simulink model "MODAL"  (R2013a)
settings: Solver=ode45  StartTime=0.0  StopTime=10.0  RelTol=1e-3
undefined symbols (not defined in the file or in its folder): f, g1, g2, J, K, L, l1, l2, R
settings Model: Creator=ciottopinton_gus  LastModifiedBy=ciottopinton_gus

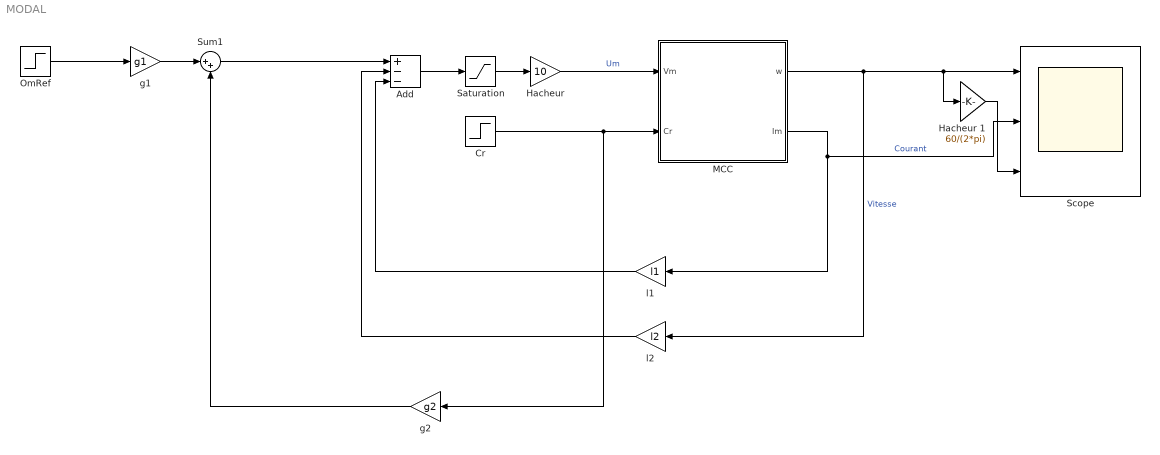
== system MODAL ==
  Add : Sum  Inputs=+--
  "Cr " : Step  Time=2  After=5  SampleTime=0
  "Hacheur " : Gain  Gain=10
  Hacheur 1 : Gain  Gain=60/(2*pi)
  MCC : Subsystem
  OmRef : Step  Time=0  After=800*2*pi/60  SampleTime=0
  Saturation : Saturate  UpperLimit=9  LowerLimit=-9
  Scope : Scope  NumInputPorts=3
      settings: YMin=-5~-5~-5  YMax=5~5~5
  Sum1 : Sum  Inputs=|++
  g1 : Gain  Gain=g1
  "g2 " : Gain  Gain=g2
  l1 : Gain  Gain=l1
  l2 : Gain  Gain=l2
  wires:
  "Hacheur "/1 -> MCC/1("Vm ")  "Um"
  Saturation/1 -> "Hacheur "/1
  Add/1 -> Saturation/1
  "Cr "/1 -> "g2 "/1, MCC/2("Cr ")
  l1/1 -> Add/3
  l2/1 -> Add/2
  MCC/2(Im) -> Scope/2, l1/1  "Courant"
  MCC/1(w) -> Scope/1, Hacheur 1/1, l2/1  "Vitesse"
  Hacheur 1/1 -> Scope/3
  OmRef/1 -> g1/1
  g1/1 -> Sum1/1
  "g2 "/1 -> Sum1/2
  Sum1/1 -> Add/1

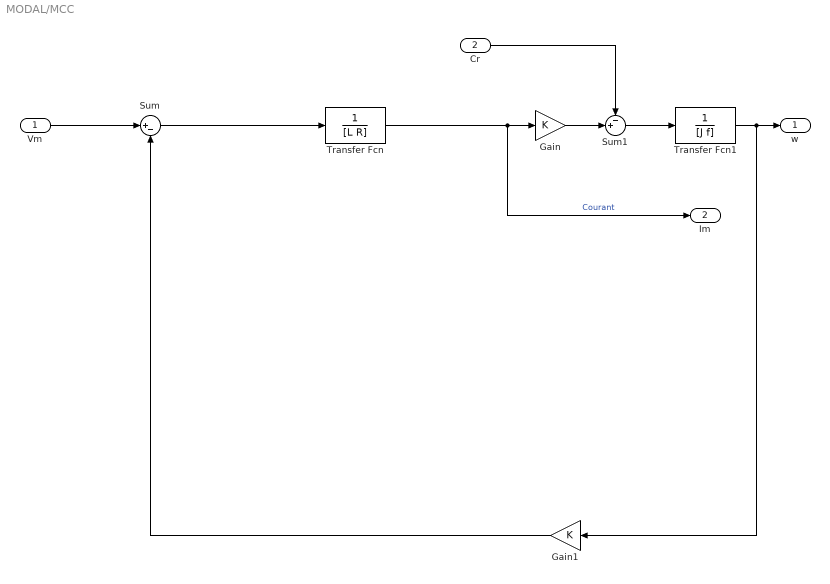
== system MODAL/MCC ==
  "Vm " : Inport
  "Cr " : Inport  Port=2
  Gain : Gain  Gain=K
  Gain1 : Gain  Gain=K
  Sum : Sum  Inputs=|+-
  Sum1 : Sum  Inputs=-+|
  Transfer Fcn : TransferFcn  Denominator=[L R]
  Transfer Fcn1 : TransferFcn  Denominator=[J f]
  w : Outport
  Im : Outport  Port=2
  wires:
  "Vm "/1 -> Sum/1
  Gain/1 -> Sum1/2
  "Cr "/1 -> Sum1/1
  Sum1/1 -> Transfer Fcn1/1
  Transfer Fcn1/1 -> Gain1/1, w/1
  Gain1/1 -> Sum/2
  Transfer Fcn/1 -> Im/1, Gain/1  "Courant"
  Sum/1 -> Transfer Fcn/1
